simulink library "Shading_Control"  (R2018b)
settings: Solver=ode45  StartTime=0.0  StopTime=10.0  RelTol=1e-3  EnableMultiTasking=on
libraries: simulink x1
settings Model: Creator=lena.frank  LastModifiedBy=P41573
settings DataIOCC: LimitDataPoints=on  SaveFormat=Array  SignalLoggingSaveFormat=ModelDataLogs
settings OptimizationCC: ExpressionDepthLimit=2147483647  LifeSpan=inf
settings DebuggingCC: UnderspecifiedInitializationDetection=Classic  MergeDetectMultiDrivingBlocksExec=none  SolverPrmCheckMsg=warning  FcnCallInpInsideContextMsg=warning  StateNameClashWarn=warning  SFUnexpectedBacktrackingDiag=warning  SFNoUnconditionalDefaultTransitionDiag=warning  SFExecutionAtInitializationDiag=none
settings HardwareCC: ProdBitPerPointer=32  ProdBitPerSizeT=32  ProdBitPerPtrDiffT=32  ProdLargestAtomicFloat=None  ProdIntDivRoundTo=Undefined  ProdEndianess=Unspecified  ProdWordSize=32  ProdHWDeviceType=32-bit Generic
settings ModelReferenceCC: PropagateSignalLabelsOutOfModel=off
settings SFSimCC: SimUseLocalCustomCode=off
settings RTWCC: RTWUseLocalCustomCode=off
settings CodeAppCC: StateflowObjectComments=on
settings GRTTargetCC: TargetLangStandard=C89/C90 (ANSI)  GeneratePreprocessorConditionals=Disable all  CombineOutputUpdateFcns=off  GRTInterface=on
settings ConfigComp: CovMetricSettings=dw  CovHtmlReporting=on  CovSaveCumulativeToWorkspaceVar=on  CovSaveSingleToWorkspaceVar=on  CovExternalEMLEnable=off

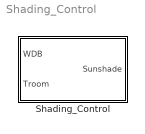
== system Shading_Control ==
  Shading_Control : Subsystem  mask(Shading Control){TroomShadeOn=23.8, TroomShadeOff=22.8, SolarShadeOn=300, SolarShadeOff=200, max_shade=1}
      mask prompts: TroomShadeOn "Room temperature to switch shading on in °C"; TroomShadeOff "Room temperature to switch shading off in °C"; SolarShadeOn "Solar radiation to switch shading on in W/m²"; SolarShadeOff "Solar radiation to switch shading off in W/m²"; max_shade "Maximum value for Sunshade"
      mask help:
      | Active the Sunshade of a window when:
      | + room temperature is above shading temperture
      | + outdoor ambient temperature is above 10°C
      | + solar radiation is above 300 W/m²
      | The solar gains of a window is:
      | SolarGain = LightTransmittance * WindowSurface
      |                     * SolarRadiation * (1 - Sunshade)
      mask TypeOptions TroomShadeOn: Hyst_Troom/OnSwitchValue
      mask TypeOptions TroomShadeOff: Hyst_Troom/OffSwitchValue
      mask TypeOptions SolarShadeOn: Hsyt_Solar/OnSwitchValue
      mask TypeOptions SolarShadeOff: Hsyt_Solar/OffSwitchValue
      mask TypeOptions max_shade: Saturation/UpperLimit
      mask Display:
      | plot(0,-5,100,95,...
      |     [70,60,60,70,80,90,90,80,70],[90,80,70,60,60,70,80,90,90],...
      |     [75,75],[91,95],[75,75],[52,58],[58,52],[75,75],...
      |     [98,91],[75,75],[63,58],[63,57],[92,86],[92,87],...
      |     [63,58],[85,92],[92,86],[57,64], ...
      |     [10,20,30,37,41,48,50,10],[51,53,53,51,45,31,20,51],...
      |     [33,30],[0,35])

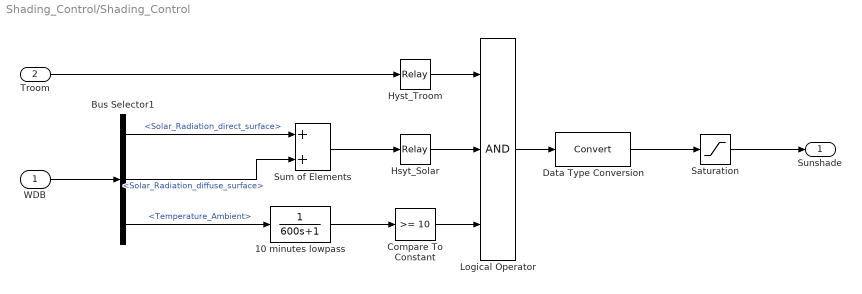
== system Shading_Control/Shading_Control ==
  WDB : Inport
  Troom : Inport  Port=2
  10 minutes lowpass : TransferFcn  Denominator=[600 1]
  Bus Selector1 : BusSelector  OutputSignals=Solar_Radiation_direct_surface,Solar_Radiation_diffuse_surface,Temperature_Ambient
  Compare To Constant : simulink/Logic and Bit Operations/Compare To Constant  relop=>=  const=10  OutDataTypeStr=uint8
  Data Type Conversion : DataTypeConversion
  Hsyt_Solar : Relay  OnSwitchValue=SolarShadeOn  OffSwitchValue=SolarShadeOff  OutDataTypeStr=uint8
  Hyst_Troom : Relay  OnSwitchValue=TroomShadeOn  OffSwitchValue=TroomShadeOff  OutDataTypeStr=uint8
  Logical Operator : Logic  Inputs=3  AllPortsSameDT=off  OutDataTypeStr=boolean
  Saturation : Saturate  UpperLimit=max_shade  LowerLimit=0
  Sum of Elements : Sum  Inputs=2
  Sunshade : Outport
  wires:
  Bus Selector1/1 -> Sum of Elements/1  "<Solar_Radiation_direct_surface>"
  10 minutes lowpass/1 -> Compare To Constant/1
  Sum of Elements/1 -> Hsyt_Solar/1
  Hsyt_Solar/1 -> Logical Operator/2
  Compare To Constant/1 -> Logical Operator/3
  Troom/1 -> Hyst_Troom/1
  WDB/1 -> Bus Selector1/1
  Hyst_Troom/1 -> Logical Operator/1
  Logical Operator/1 -> Data Type Conversion/1
  Data Type Conversion/1 -> Saturation/1
  Saturation/1 -> Sunshade/1
  Bus Selector1/2 -> Sum of Elements/2  "<Solar_Radiation_diffuse_surface>"
  Bus Selector1/3 -> 10 minutes lowpass/1  "<Temperature_Ambient>"
